simulink model "case5"  (R2024b)
settings: Solver=FixedStepAuto  StartTime=0  StopTime=1  FixedStep=1e-7  RelTol=1e-3
values from neighbouring files (symbols this model uses):
  SG_D_1_D = 0.01056    [IEEE9_case_parameters.m]    (also in case1_parameters.m; case2_parameters.m; case3_parameters.m; case4_parameters.m)
  SG_D_1_EnableSaturation = 0    [IEEE9_case_parameters.m]    (also in case1_parameters.m; case2_parameters.m; case3_parameters.m; case4_parameters.m)
  SG_D_1_f0 = 60    [IEEE9_case_parameters.m]    (also in case1_parameters.m; case2_parameters.m; case3_parameters.m; case4_parameters.m)
  SG_D_1_H = 7.5    [IEEE9_case_parameters.m]    (also in case1_parameters.m; case2_parameters.m; case3_parameters.m; case4_parameters.m)
  SG_D_1_K_A = 20    [IEEE9_case_parameters.m]    (also in case1_parameters.m; case2_parameters.m; case3_parameters.m; case4_parameters.m)
  SG_D_1_K_E = 1.000000e+1    (= 10)    [IEEE9_case_parameters.m]    (also in case1_parameters.m; case2_parameters.m; case3_parameters.m; case4_parameters.m)
  SG_D_1_K_F = 2.363    [IEEE9_case_parameters.m]    (also in case1_parameters.m; case2_parameters.m; case3_parameters.m; case4_parameters.m)
  SG_D_1_K_s = 0.5    [IEEE9_case_parameters.m]    (also in case1_parameters.m = 5; case2_parameters.m = 5; case3_parameters.m = 5; case4_parameters.m = 5)
  SG_D_1_R_a = 0.001088    [IEEE9_case_parameters.m]    (also in case1_parameters.m; case2_parameters.m; case3_parameters.m; case4_parameters.m)
  SG_D_1_S_A = 1    [IEEE9_case_parameters.m]    (also in case1_parameters.m; case2_parameters.m; case3_parameters.m; case4_parameters.m)
  SG_D_1_S_B = 0.103    [IEEE9_case_parameters.m]    (also in case1_parameters.m; case2_parameters.m; case3_parameters.m; case4_parameters.m)
  SG_D_1_S_N = 10.659857    [IEEE9_case_parameters.m]    (also in case1_parameters.m; case2_parameters.m; case3_parameters.m; case4_parameters.m)
  SG_D_1_SpeedPara = 200    [IEEE9_case_parameters.m]    (also in case1_parameters.m; case2_parameters.m; case3_parameters.m; case4_parameters.m)
  SG_D_1_T_0 = 0.720173    [IEEE9_case_parameters.m]    (also in case1_parameters.m = 0.755522; case2_parameters.m = 0.808931; case3_parameters.m = 0.869402; case4_parameters.m = 0.729316)
  SG_D_1_T_1 = 0.3    [IEEE9_case_parameters.m]    (also in case1_parameters.m; case2_parameters.m; case3_parameters.m; case4_parameters.m)
  SG_D_1_T_2 = 0.05    [IEEE9_case_parameters.m]    (also in case1_parameters.m; case2_parameters.m; case3_parameters.m; case4_parameters.m)
  SG_D_1_T_3 = 0.02    [IEEE9_case_parameters.m]    (also in case1_parameters.m; case2_parameters.m; case3_parameters.m; case4_parameters.m)
  SG_D_1_T_4 = 0.005    [IEEE9_case_parameters.m]    (also in case1_parameters.m; case2_parameters.m; case3_parameters.m; case4_parameters.m)
  SG_D_1_T_A = 0.02    [IEEE9_case_parameters.m]    (also in case1_parameters.m; case2_parameters.m; case3_parameters.m; case4_parameters.m)
  SG_D_1_T_dd = 8.000000e+0    (= 8)    [IEEE9_case_parameters.m]    (also in case1_parameters.m; case2_parameters.m; case3_parameters.m; case4_parameters.m)
  SG_D_1_T_ddd = 0.04    [IEEE9_case_parameters.m]    (also in case1_parameters.m; case2_parameters.m; case3_parameters.m; case4_parameters.m)
  SG_D_1_T_E = 0.314    [IEEE9_case_parameters.m]    (also in case1_parameters.m; case2_parameters.m; case3_parameters.m; case4_parameters.m)
  SG_D_1_T_F = 0.35    [IEEE9_case_parameters.m]    (also in case1_parameters.m; case2_parameters.m; case3_parameters.m; case4_parameters.m)
  SG_D_1_T_qd = 0.8    [IEEE9_case_parameters.m]    (also in case1_parameters.m; case2_parameters.m; case3_parameters.m; case4_parameters.m)
  SG_D_1_T_qdd = 0.02    [IEEE9_case_parameters.m]    (also in case1_parameters.m; case2_parameters.m; case3_parameters.m; case4_parameters.m)
  SG_D_1_T_speed = 0.1    [IEEE9_case_parameters.m]    (also in case1_parameters.m = 200; case2_parameters.m = 200; case3_parameters.m = 200; case4_parameters.m = 200)
  SG_D_1_T_w = 0.5    [IEEE9_case_parameters.m]    (also in case1_parameters.m; case2_parameters.m; case3_parameters.m; case4_parameters.m)
  SG_D_1_V_ref = 1.990276    [IEEE9_case_parameters.m]    (also in case1_parameters.m = 2.042296; case2_parameters.m = 2.051388; case3_parameters.m = 2.089584; case4_parameters.m = 2.01845)
  SG_D_1_w_ref = 376.991118    [IEEE9_case_parameters.m]    (also in case1_parameters.m; case2_parameters.m; case3_parameters.m; case4_parameters.m)
  SG_D_1_wb = 6.000000e+1    (= 60)    [IEEE9_case_parameters.m]    (also in case1_parameters.m; case2_parameters.m; case3_parameters.m; case4_parameters.m)
  SG_D_1_x_d = 1.9    [IEEE9_case_parameters.m]    (also in case1_parameters.m; case2_parameters.m; case3_parameters.m; case4_parameters.m)
  SG_D_1_x_dd = 0.302    [IEEE9_case_parameters.m]    (also in case1_parameters.m; case2_parameters.m; case3_parameters.m; case4_parameters.m)
  SG_D_1_x_ddd = 0.204    [IEEE9_case_parameters.m]    (also in case1_parameters.m; case2_parameters.m; case3_parameters.m; case4_parameters.m)
  SG_D_1_x_l = 0.05    [IEEE9_case_parameters.m]    (also in case1_parameters.m; case2_parameters.m; case3_parameters.m; case4_parameters.m)
  SG_D_1_x_q = 1.3    [IEEE9_case_parameters.m]    (also in case1_parameters.m; case2_parameters.m; case3_parameters.m; case4_parameters.m)
  SG_D_1_x_qd = 0.5    [IEEE9_case_parameters.m]    (also in case1_parameters.m; case2_parameters.m; case3_parameters.m; case4_parameters.m)
  SG_D_1_x_qdd = 0.3    [IEEE9_case_parameters.m]    (also in case1_parameters.m; case2_parameters.m; case3_parameters.m; case4_parameters.m)
  SG_D_2_D = 0.02    [IEEE9_case_parameters.m]    (also in case1_parameters.m; case2_parameters.m; case3_parameters.m; case4_parameters.m)
  SG_D_2_EnableSaturation = 0    [IEEE9_case_parameters.m]    (also in case1_parameters.m; case2_parameters.m; case3_parameters.m; case4_parameters.m)
  SG_D_2_f0 = 60    [IEEE9_case_parameters.m]    (also in case1_parameters.m; case2_parameters.m; case3_parameters.m; case4_parameters.m)
  SG_D_2_H = 8.000000e+0    (= 8)    [IEEE9_case_parameters.m]    (also in case1_parameters.m; case2_parameters.m; case3_parameters.m; case4_parameters.m)
  SG_D_2_K_A = 20    [IEEE9_case_parameters.m]    (also in case1_parameters.m; case2_parameters.m; case3_parameters.m; case4_parameters.m)
  SG_D_2_K_E = 1.000000e+1    (= 10)    [IEEE9_case_parameters.m]    (also in case1_parameters.m; case2_parameters.m; case3_parameters.m; case4_parameters.m)
  SG_D_2_K_F = 2.363    [IEEE9_case_parameters.m]    (also in case1_parameters.m; case2_parameters.m; case3_parameters.m; case4_parameters.m)
  SG_D_2_K_s = 0.5    [IEEE9_case_parameters.m]    (also in case1_parameters.m = 4; case2_parameters.m = 4; case3_parameters.m = 4; case4_parameters.m = 4)
  SG_D_2_R_a = 0.001088    [IEEE9_case_parameters.m]    (also in case1_parameters.m; case2_parameters.m; case3_parameters.m; case4_parameters.m)
  SG_D_2_S_A = 1    [IEEE9_case_parameters.m]    (also in case1_parameters.m; case2_parameters.m; case3_parameters.m; case4_parameters.m)
  SG_D_2_S_B = 0.103    [IEEE9_case_parameters.m]    (also in case1_parameters.m; case2_parameters.m; case3_parameters.m; case4_parameters.m)
  SG_D_2_S_N = 10.659857    [IEEE9_case_parameters.m]    (also in case1_parameters.m; case2_parameters.m; case3_parameters.m; case4_parameters.m)
  SG_D_2_SpeedPara = 200    [IEEE9_case_parameters.m]    (also in case1_parameters.m; case2_parameters.m; case3_parameters.m; case4_parameters.m)
  SG_D_2_T_0 = 1.632913    [IEEE9_case_parameters.m]    (also in case1_parameters.m = 1.632925; case2_parameters.m = 1.632915; case3_parameters.m = 1.632914; case4_parameters.m = 1.632927)
  SG_D_2_T_1 = 0.2    [IEEE9_case_parameters.m]    (also in case1_parameters.m; case2_parameters.m; case3_parameters.m; case4_parameters.m)
  SG_D_2_T_2 = 0.05    [IEEE9_case_parameters.m]    (also in case1_parameters.m; case2_parameters.m; case3_parameters.m; case4_parameters.m)
  SG_D_2_T_3 = 0.02    [IEEE9_case_parameters.m]    (also in case1_parameters.m; case2_parameters.m; case3_parameters.m; case4_parameters.m)
  SG_D_2_T_4 = 0.005    [IEEE9_case_parameters.m]    (also in case1_parameters.m; case2_parameters.m; case3_parameters.m; case4_parameters.m)
  SG_D_2_T_A = 0.02    [IEEE9_case_parameters.m]    (also in case1_parameters.m; case2_parameters.m; case3_parameters.m; case4_parameters.m)
  SG_D_2_T_dd = 7.9    [IEEE9_case_parameters.m]    (also in case1_parameters.m; case2_parameters.m; case3_parameters.m; case4_parameters.m)
  SG_D_2_T_ddd = 0.04    [IEEE9_case_parameters.m]    (also in case1_parameters.m; case2_parameters.m; case3_parameters.m; case4_parameters.m)
  SG_D_2_T_E = 0.314    [IEEE9_case_parameters.m]    (also in case1_parameters.m; case2_parameters.m; case3_parameters.m; case4_parameters.m)
  SG_D_2_T_F = 0.35    [IEEE9_case_parameters.m]    (also in case1_parameters.m; case2_parameters.m; case3_parameters.m; case4_parameters.m)
  SG_D_2_T_qd = 0.8    [IEEE9_case_parameters.m]    (also in case1_parameters.m; case2_parameters.m; case3_parameters.m; case4_parameters.m)
  SG_D_2_T_qdd = 0.015    [IEEE9_case_parameters.m]    (also in case1_parameters.m; case2_parameters.m; case3_parameters.m; case4_parameters.m)
  SG_D_2_T_speed = 0.1    [IEEE9_case_parameters.m]    (also in case1_parameters.m = 150; case2_parameters.m = 150; case3_parameters.m = 150; case4_parameters.m = 150)
  SG_D_2_T_w = 0.35    [IEEE9_case_parameters.m]    (also in case1_parameters.m; case2_parameters.m; case3_parameters.m; case4_parameters.m)
  SG_D_2_V_ref = 2.58547    [IEEE9_case_parameters.m]    (also in case1_parameters.m = 2.597896; case2_parameters.m = 2.587136; case3_parameters.m = 2.586042; case4_parameters.m = 2.599679)
  SG_D_2_w_ref = 376.991118    [IEEE9_case_parameters.m]    (also in case1_parameters.m; case2_parameters.m; case3_parameters.m; case4_parameters.m)
  SG_D_2_wb = 6.000000e+1    (= 60)    [IEEE9_case_parameters.m]    (also in case1_parameters.m; case2_parameters.m; case3_parameters.m; case4_parameters.m)
  SG_D_2_x_d = 1.8    [IEEE9_case_parameters.m]    (also in case1_parameters.m; case2_parameters.m; case3_parameters.m; case4_parameters.m)
  SG_D_2_x_dd = 0.302    [IEEE9_case_parameters.m]    (also in case1_parameters.m; case2_parameters.m; case3_parameters.m; case4_parameters.m)
  SG_D_2_x_ddd = 0.204    [IEEE9_case_parameters.m]    (also in case1_parameters.m; case2_parameters.m; case3_parameters.m; case4_parameters.m)
  SG_D_2_x_l = 0.05    [IEEE9_case_parameters.m]    (also in case1_parameters.m; case2_parameters.m; case3_parameters.m; case4_parameters.m)
  SG_D_2_x_q = 1.25    [IEEE9_case_parameters.m]    (also in case1_parameters.m; case2_parameters.m; case3_parameters.m; case4_parameters.m)
  SG_D_2_x_qd = 0.5    [IEEE9_case_parameters.m]    (also in case1_parameters.m; case2_parameters.m; case3_parameters.m; case4_parameters.m)
  SG_D_2_x_qdd = 0.3    [IEEE9_case_parameters.m]    (also in case1_parameters.m; case2_parameters.m; case3_parameters.m; case4_parameters.m)
  SG_D_3_D = 0.02    [IEEE9_case_parameters.m]    (also in case1_parameters.m; case2_parameters.m; case3_parameters.m; case4_parameters.m)
  SG_D_3_EnableSaturation = 0    [IEEE9_case_parameters.m]    (also in case1_parameters.m; case2_parameters.m; case3_parameters.m; case4_parameters.m)
  SG_D_3_f0 = 60    [IEEE9_case_parameters.m]    (also in case1_parameters.m; case2_parameters.m; case3_parameters.m; case4_parameters.m)
  SG_D_3_H = 7.7    [IEEE9_case_parameters.m]    (also in case1_parameters.m; case2_parameters.m; case3_parameters.m; case4_parameters.m)
  SG_D_3_K_A = 20    [IEEE9_case_parameters.m]    (also in case1_parameters.m; case2_parameters.m; case3_parameters.m; case4_parameters.m)
  SG_D_3_K_E = 1.000000e+1    (= 10)    [IEEE9_case_parameters.m]    (also in case1_parameters.m; case2_parameters.m; case3_parameters.m; case4_parameters.m)
  SG_D_3_K_F = 2.363    [IEEE9_case_parameters.m]    (also in case1_parameters.m; case2_parameters.m; case3_parameters.m; case4_parameters.m)
  SG_D_3_K_s = 0.2    [IEEE9_case_parameters.m]    (also in case1_parameters.m = 2; case2_parameters.m = 2; case3_parameters.m = 2; case4_parameters.m = 2)
  SG_D_3_R_a = 0.001088    [IEEE9_case_parameters.m]    (also in case1_parameters.m; case2_parameters.m; case3_parameters.m; case4_parameters.m)
  SG_D_3_S_A = 1    [IEEE9_case_parameters.m]    (also in case1_parameters.m; case2_parameters.m; case3_parameters.m; case4_parameters.m)
  SG_D_3_S_B = 0.103    [IEEE9_case_parameters.m]    (also in case1_parameters.m; case2_parameters.m; case3_parameters.m; case4_parameters.m)
  SG_D_3_S_N = 10.659857    [IEEE9_case_parameters.m]    (also in case1_parameters.m; case2_parameters.m; case3_parameters.m; case4_parameters.m)
  SG_D_3_SpeedPara = 200    [IEEE9_case_parameters.m]    (also in case1_parameters.m; case2_parameters.m; case3_parameters.m; case4_parameters.m)
  SG_D_3_T_0 = 0.850788    [IEEE9_case_parameters.m]    (also in case1_parameters.m = 0.850786; case2_parameters.m = 0.850787; case3_parameters.m; case4_parameters.m = 0.850786)
  SG_D_3_T_1 = 0.2    [IEEE9_case_parameters.m]    (also in case1_parameters.m; case2_parameters.m; case3_parameters.m; case4_parameters.m)
  SG_D_3_T_2 = 0.05    [IEEE9_case_parameters.m]    (also in case1_parameters.m; case2_parameters.m; case3_parameters.m; case4_parameters.m)
  SG_D_3_T_3 = 0.02    [IEEE9_case_parameters.m]    (also in case1_parameters.m; case2_parameters.m; case3_parameters.m; case4_parameters.m)
  SG_D_3_T_4 = 0.005    [IEEE9_case_parameters.m]    (also in case1_parameters.m; case2_parameters.m; case3_parameters.m; case4_parameters.m)
  SG_D_3_T_A = 0.02    [IEEE9_case_parameters.m]    (also in case1_parameters.m; case2_parameters.m; case3_parameters.m; case4_parameters.m)
  SG_D_3_T_dd = 8.1    [IEEE9_case_parameters.m]    (also in case1_parameters.m; case2_parameters.m; case3_parameters.m; case4_parameters.m)
  SG_D_3_T_ddd = 0.04    [IEEE9_case_parameters.m]    (also in case1_parameters.m; case2_parameters.m; case3_parameters.m; case4_parameters.m)
  SG_D_3_T_E = 0.314    [IEEE9_case_parameters.m]    (also in case1_parameters.m; case2_parameters.m; case3_parameters.m; case4_parameters.m)
  SG_D_3_T_F = 0.35    [IEEE9_case_parameters.m]    (also in case1_parameters.m; case2_parameters.m; case3_parameters.m; case4_parameters.m)
  SG_D_3_T_qd = 0.8    [IEEE9_case_parameters.m]    (also in case1_parameters.m; case2_parameters.m; case3_parameters.m; case4_parameters.m)
  SG_D_3_T_qdd = 0.015    [IEEE9_case_parameters.m]    (also in case1_parameters.m; case2_parameters.m; case3_parameters.m; case4_parameters.m)
  SG_D_3_T_speed = 0.1    [IEEE9_case_parameters.m]    (also in case1_parameters.m = 180; case2_parameters.m = 180; case3_parameters.m = 180; case4_parameters.m = 180)
  SG_D_3_T_w = 0.4    [IEEE9_case_parameters.m]    (also in case1_parameters.m; case2_parameters.m; case3_parameters.m; case4_parameters.m)
  SG_D_3_V_ref = 1.892727    [IEEE9_case_parameters.m]    (also in case1_parameters.m = 1.906439; case2_parameters.m = 1.895535; case3_parameters.m = 1.892105; case4_parameters.m = 1.906598)
  SG_D_3_w_ref = 376.991118    [IEEE9_case_parameters.m]    (also in case1_parameters.m; case2_parameters.m; case3_parameters.m; case4_parameters.m)
  SG_D_3_wb = 6.000000e+1    (= 60)    [IEEE9_case_parameters.m]    (also in case1_parameters.m; case2_parameters.m; case3_parameters.m; case4_parameters.m)
  SG_D_3_x_d = 1.85    [IEEE9_case_parameters.m]    (also in case1_parameters.m; case2_parameters.m; case3_parameters.m; case4_parameters.m)
  SG_D_3_x_dd = 0.302    [IEEE9_case_parameters.m]    (also in case1_parameters.m; case2_parameters.m; case3_parameters.m; case4_parameters.m)
  SG_D_3_x_ddd = 0.204    [IEEE9_case_parameters.m]    (also in case1_parameters.m; case2_parameters.m; case3_parameters.m; case4_parameters.m)
  SG_D_3_x_l = 0.05    [IEEE9_case_parameters.m]    (also in case1_parameters.m; case2_parameters.m; case3_parameters.m; case4_parameters.m)
  SG_D_3_x_q = 1.2    [IEEE9_case_parameters.m]    (also in case1_parameters.m; case2_parameters.m; case3_parameters.m; case4_parameters.m)
  SG_D_3_x_qd = 0.5    [IEEE9_case_parameters.m]    (also in case1_parameters.m; case2_parameters.m; case3_parameters.m; case4_parameters.m)
  SG_D_3_x_qdd = 0.3    [IEEE9_case_parameters.m]    (also in case1_parameters.m; case2_parameters.m; case3_parameters.m; case4_parameters.m)
(part 4 of 12)

== system case5/AC_1/d_vq_bus_7_block ==
  note: d_vq_bus_7 in case5
      | $2106.09563369148\,\mathrm{iq}_{\mathrm{bus},7}-376.991118430775\,\mathrm{vd}_{\mathrm{bus},7}$
      | Automatically generated on 2025-10-31 19:13:58 .
  Alge_iq_bus_7_45bb2 : Inport
  State_vd_bus_7_3739f : Inport  Port=2
  Constant_2106.09563369148_ba6a5 : Constant  Value=2106.09563369148
  Constant_376.991118430775_2faa8 : Constant  Value=376.991118430775
  Product_6eb21 : Product
  Product_90d6e : Product
  Subtract_950c2 : Sum  Inputs=+-
  Blockout_d_vq_bus_7_12864 : Outport
  wires:
  Constant_2106.09563369148_ba6a5/1 -> Product_6eb21/1
  Product_90d6e/1 -> Subtract_950c2/2
  Alge_iq_bus_7_45bb2/1 -> Product_6eb21/2
  Constant_376.991118430775_2faa8/1 -> Product_90d6e/1
  Subtract_950c2/1 -> Blockout_d_vq_bus_7_12864/1
  State_vd_bus_7_3739f/1 -> Product_90d6e/2
  Product_6eb21/1 -> Subtract_950c2/1

== system case5/AC_1/d_vq_bus_8_block ==
  note: d_vq_bus_8 in case5
      | $1657.10381727813\,\mathrm{iq}_{\mathrm{bus},8}-376.991118430775\,\mathrm{vd}_{\mathrm{bus},8}$
      | Automatically generated on 2025-10-31 19:14:00 .
  Alge_iq_bus_8_1b1c2 : Inport
  State_vd_bus_8_d6cf7 : Inport  Port=2
  Constant_1657.10381727813_ee9d3 : Constant  Value=1657.10381727813
  Constant_376.991118430775_c08d9 : Constant  Value=376.991118430775
  Product_2c011 : Product
  Product_4bb21 : Product
  Subtract_80bfc : Sum  Inputs=+-
  Blockout_d_vq_bus_8_57dfd : Outport
  wires:
  Constant_1657.10381727813_ee9d3/1 -> Product_2c011/1
  Constant_376.991118430775_c08d9/1 -> Product_4bb21/1
  Alge_iq_bus_8_1b1c2/1 -> Product_2c011/2
  State_vd_bus_8_d6cf7/1 -> Product_4bb21/2
  Product_2c011/1 -> Subtract_80bfc/1
  Product_4bb21/1 -> Subtract_80bfc/2
  Subtract_80bfc/1 -> Blockout_d_vq_bus_8_57dfd/1

== system case5/AC_1/d_vq_bus_9_block ==
  note: d_vq_bus_9 in case5
      | $1564.27849971276\,\mathrm{iq}_{\mathrm{bus},9}-376.991118430775\,\mathrm{vd}_{\mathrm{bus},9}$
      | Automatically generated on 2025-10-31 19:14:02 .
  Alge_iq_bus_9_3d507 : Inport
  State_vd_bus_9_5d984 : Inport  Port=2
  Constant_1564.27849971276_97533 : Constant  Value=1564.27849971276
  Constant_376.991118430775_b4458 : Constant  Value=376.991118430775
  Product_0f672 : Product
  Product_b1dd5 : Product
  Subtract_083c6 : Sum  Inputs=+-
  Blockout_d_vq_bus_9_906de : Outport
  wires:
  Constant_1564.27849971276_97533/1 -> Product_0f672/1
  Constant_376.991118430775_b4458/1 -> Product_b1dd5/1
  Alge_iq_bus_9_3d507/1 -> Product_0f672/2
  State_vd_bus_9_5d984/1 -> Product_b1dd5/2
  Product_0f672/1 -> Subtract_083c6/1
  Product_b1dd5/1 -> Subtract_083c6/2
  Subtract_083c6/1 -> Blockout_d_vq_bus_9_906de/1

== system case5/AC_1/id_bus_1_block ==
  note: id_bus_1 in case5
      | $\mathrm{id}_{\mathrm{SG},D,1}-\mathrm{id}_{\mathrm{line},1,4}$
      | Automatically generated on 2025-10-31 19:14:43 .
  Input_id_SG_D_1_9c228 : Inport
  State_id_line_1_4_23de7 : Inport  Port=2
  Subtract_cb11a : Sum  Inputs=+-
  Blockout_id_bus_1_91a25 : Outport
  wires:
  Input_id_SG_D_1_9c228/1 -> Subtract_cb11a/1
  State_id_line_1_4_23de7/1 -> Subtract_cb11a/2
  Subtract_cb11a/1 -> Blockout_id_bus_1_91a25/1

== system case5/AC_1/id_bus_2_block ==
  note: id_bus_2 in case5
      | $\mathrm{id}_{\mathrm{SG},D,2}+\mathrm{id}_{\mathrm{line},8,2}$
      | Automatically generated on 2025-10-31 19:14:45 .
  Input_id_SG_D_2_cb453 : Inport
  State_id_line_8_2_49dbc : Inport  Port=2
  Add_a3873 : Sum
  Blockout_id_bus_2_c40f0 : Outport
  wires:
  Input_id_SG_D_2_cb453/1 -> Add_a3873/1
  State_id_line_8_2_49dbc/1 -> Add_a3873/2
  Add_a3873/1 -> Blockout_id_bus_2_c40f0/1

== system case5/AC_1/id_bus_3_block ==
  note: id_bus_3 in case5
      | $\mathrm{id}_{\mathrm{SG},D,3}-\mathrm{id}_{\mathrm{line},3,6}$
      | Automatically generated on 2025-10-31 19:14:48 .
  Input_id_SG_D_3_99f83 : Inport
  State_id_line_3_6_1713b : Inport  Port=2
  Subtract_3e534 : Sum  Inputs=+-
  Blockout_id_bus_3_bec8f : Outport
  wires:
  Input_id_SG_D_3_99f83/1 -> Subtract_3e534/1
  State_id_line_3_6_1713b/1 -> Subtract_3e534/2
  Subtract_3e534/1 -> Blockout_id_bus_3_bec8f/1

== system case5/AC_1/id_bus_4_block ==
  note: id_bus_4 in case5
      | $\mathrm{id}_{\mathrm{line},1,4}-\mathrm{id}_{\mathrm{line},4,5}+\mathrm{id}_{\mathrm{line},9,4}$
      | Automatically generated on 2025-10-31 19:14:50 .
  State_id_line_1_4_47296 : Inport
  State_id_line_4_5_4344a : Inport  Port=2
  State_id_line_9_4_2502b : Inport  Port=3
  Add_be097 : Sum
  Subtract_45d26 : Sum  Inputs=+-
  Blockout_id_bus_4_70fca : Outport
  wires:
  State_id_line_9_4_2502b/1 -> Add_be097/2
  State_id_line_1_4_47296/1 -> Subtract_45d26/1
  State_id_line_4_5_4344a/1 -> Subtract_45d26/2
  Subtract_45d26/1 -> Add_be097/1
  Add_be097/1 -> Blockout_id_bus_4_70fca/1

== system case5/AC_1/id_bus_5_block ==
  note: id_bus_5 in case5
      | $\mathrm{id}_{\mathrm{line},4,5}-\mathrm{id}_{\mathrm{load},5}-\mathrm{id}_{\mathrm{line},5,6}$
      | Automatically generated on 2025-10-31 19:14:52 .
  State_id_load_5_d4ed3 : Inport
  State_id_line_4_5_425cc : Inport  Port=2
  State_id_line_5_6_e79c9 : Inport  Port=3
  Add_efccb : Sum
  Constant_-1_cbbea : Constant  Value=-1
  Product_350a7 : Product
  Subtract_95ac5 : Sum  Inputs=+-
  Blockout_id_bus_5_e7f75 : Outport
  wires:
  Subtract_95ac5/1 -> Blockout_id_bus_5_e7f75/1
  State_id_line_4_5_425cc/1 -> Add_efccb/2
  Constant_-1_cbbea/1 -> Product_350a7/1
  Add_efccb/1 -> Subtract_95ac5/1
  State_id_load_5_d4ed3/1 -> Product_350a7/2
  Product_350a7/1 -> Add_efccb/1
  State_id_line_5_6_e79c9/1 -> Subtract_95ac5/2

== system case5/AC_1/id_bus_6_block ==
  note: id_bus_6 in case5
      | $\mathrm{id}_{\mathrm{line},3,6}+\mathrm{id}_{\mathrm{line},5,6}-\mathrm{id}_{\mathrm{line},6,7}$
      | Automatically generated on 2025-10-31 19:14:54 .
  State_id_line_3_6_811b8 : Inport
  State_id_line_5_6_98abd : Inport  Port=2
  State_id_line_6_7_21130 : Inport  Port=3
  Add_d4af5 : Sum
  Subtract_01d0a : Sum  Inputs=+-
  Blockout_id_bus_6_b6b8c : Outport
  wires:
  State_id_line_6_7_21130/1 -> Subtract_01d0a/2
  State_id_line_3_6_811b8/1 -> Add_d4af5/1
  State_id_line_5_6_98abd/1 -> Add_d4af5/2
  Add_d4af5/1 -> Subtract_01d0a/1
  Subtract_01d0a/1 -> Blockout_id_bus_6_b6b8c/1

== system case5/AC_1/id_bus_7_block ==
  note: id_bus_7 in case5
      | $\mathrm{id}_{\mathrm{line},6,7}-\mathrm{id}_{\mathrm{load},7}-\mathrm{id}_{\mathrm{line},7,8}$
      | Automatically generated on 2025-10-31 19:14:56 .
  State_id_load_7_7bf08 : Inport
  State_id_line_6_7_06d30 : Inport  Port=2
  State_id_line_7_8_80602 : Inport  Port=3
  Add_eed5a : Sum
  Constant_-1_70b3b : Constant  Value=-1
  Product_29b3c : Product
  Subtract_43355 : Sum  Inputs=+-
  Blockout_id_bus_7_23be7 : Outport
  wires:
  Subtract_43355/1 -> Blockout_id_bus_7_23be7/1
  State_id_line_6_7_06d30/1 -> Add_eed5a/2
  Constant_-1_70b3b/1 -> Product_29b3c/1
  Add_eed5a/1 -> Subtract_43355/1
  State_id_load_7_7bf08/1 -> Product_29b3c/2
  Product_29b3c/1 -> Add_eed5a/1
  State_id_line_7_8_80602/1 -> Subtract_43355/2

== system case5/AC_1/id_bus_8_block ==
  note: id_bus_8 in case5
      | $\mathrm{id}_{\mathrm{line},7,8}-\mathrm{id}_{\mathrm{line},8,2}-\mathrm{id}_{\mathrm{line},8,9}$
      | Automatically generated on 2025-10-31 19:14:58 .
  State_id_line_7_8_30e25 : Inport
  State_id_line_8_2_6b72a : Inport  Port=2
  State_id_line_8_9_be4b7 : Inport  Port=3
  Subtract_2ee3c : Sum  Inputs=+-
  Subtract_46dea : Sum  Inputs=+-
  Blockout_id_bus_8_10175 : Outport
  wires:
  State_id_line_8_9_be4b7/1 -> Subtract_2ee3c/2
  State_id_line_7_8_30e25/1 -> Subtract_46dea/1
  State_id_line_8_2_6b72a/1 -> Subtract_46dea/2
  Subtract_46dea/1 -> Subtract_2ee3c/1
  Subtract_2ee3c/1 -> Blockout_id_bus_8_10175/1

== system case5/AC_1/id_bus_9_block ==
  note: id_bus_9 in case5
      | $\mathrm{id}_{\mathrm{line},8,9}-\mathrm{id}_{\mathrm{load},9}-\mathrm{id}_{\mathrm{line},9,4}$
      | Automatically generated on 2025-10-31 19:15:00 .
  State_id_load_9_599d3 : Inport
  State_id_line_8_9_6f7fd : Inport  Port=2
  State_id_line_9_4_83515 : Inport  Port=3
  Add_55017 : Sum
  Constant_-1_0a66a : Constant  Value=-1
  Product_dee9f : Product
  Subtract_f3c68 : Sum  Inputs=+-
  Blockout_id_bus_9_60bfe : Outport
  wires:
  Subtract_f3c68/1 -> Blockout_id_bus_9_60bfe/1
  State_id_line_8_9_6f7fd/1 -> Add_55017/2
  Constant_-1_0a66a/1 -> Product_dee9f/1
  Add_55017/1 -> Subtract_f3c68/1
  State_id_load_9_599d3/1 -> Product_dee9f/2
  Product_dee9f/1 -> Add_55017/1
  State_id_line_9_4_83515/1 -> Subtract_f3c68/2

== system case5/AC_1/iq_bus_1_block ==
  note: iq_bus_1 in case5
      | $\mathrm{iq}_{\mathrm{SG},D,1}-\mathrm{iq}_{\mathrm{line},1,4}$
      | Automatically generated on 2025-10-31 19:14:43 .
  Input_iq_SG_D_1_08f14 : Inport
  State_iq_line_1_4_e657d : Inport  Port=2
  Subtract_aca48 : Sum  Inputs=+-
  Blockout_iq_bus_1_da657 : Outport
  wires:
  Input_iq_SG_D_1_08f14/1 -> Subtract_aca48/1
  State_iq_line_1_4_e657d/1 -> Subtract_aca48/2
  Subtract_aca48/1 -> Blockout_iq_bus_1_da657/1

== system case5/AC_1/iq_bus_2_block ==
  note: iq_bus_2 in case5
      | $\mathrm{iq}_{\mathrm{SG},D,2}+\mathrm{iq}_{\mathrm{line},8,2}$
      | Automatically generated on 2025-10-31 19:14:46 .
  Input_iq_SG_D_2_79eaf : Inport
  State_iq_line_8_2_2ed82 : Inport  Port=2
  Add_b955d : Sum
  Blockout_iq_bus_2_efb5b : Outport
  wires:
  Input_iq_SG_D_2_79eaf/1 -> Add_b955d/1
  State_iq_line_8_2_2ed82/1 -> Add_b955d/2
  Add_b955d/1 -> Blockout_iq_bus_2_efb5b/1

== system case5/AC_1/iq_bus_3_block ==
  note: iq_bus_3 in case5
      | $\mathrm{iq}_{\mathrm{SG},D,3}-\mathrm{iq}_{\mathrm{line},3,6}$
      | Automatically generated on 2025-10-31 19:14:49 .
  Input_iq_SG_D_3_679b5 : Inport
  State_iq_line_3_6_d3a99 : Inport  Port=2
  Subtract_36106 : Sum  Inputs=+-
  Blockout_iq_bus_3_3b6b3 : Outport
  wires:
  Input_iq_SG_D_3_679b5/1 -> Subtract_36106/1
  State_iq_line_3_6_d3a99/1 -> Subtract_36106/2
  Subtract_36106/1 -> Blockout_iq_bus_3_3b6b3/1

== system case5/AC_1/iq_bus_4_block ==
  note: iq_bus_4 in case5
      | $\mathrm{iq}_{\mathrm{line},1,4}-\mathrm{iq}_{\mathrm{line},4,5}+\mathrm{iq}_{\mathrm{line},9,4}$
      | Automatically generated on 2025-10-31 19:14:51 .
  State_iq_line_1_4_c5db2 : Inport
  State_iq_line_4_5_0f8d8 : Inport  Port=2
  State_iq_line_9_4_ed85c : Inport  Port=3
  Add_38c5e : Sum
  Subtract_8af62 : Sum  Inputs=+-
  Blockout_iq_bus_4_10eb1 : Outport
  wires:
  State_iq_line_1_4_c5db2/1 -> Subtract_8af62/1
  State_iq_line_4_5_0f8d8/1 -> Subtract_8af62/2
  Subtract_8af62/1 -> Add_38c5e/1
  State_iq_line_9_4_ed85c/1 -> Add_38c5e/2
  Add_38c5e/1 -> Blockout_iq_bus_4_10eb1/1

== system case5/AC_1/iq_bus_5_block ==
  note: iq_bus_5 in case5
      | $\mathrm{iq}_{\mathrm{line},4,5}-\mathrm{iq}_{\mathrm{load},5}-\mathrm{iq}_{\mathrm{line},5,6}$
      | Automatically generated on 2025-10-31 19:14:53 .
  State_iq_load_5_13280 : Inport
  State_iq_line_4_5_a44be : Inport  Port=2
  State_iq_line_5_6_a1b62 : Inport  Port=3
  Add_5db17 : Sum
  Constant_-1_aaef8 : Constant  Value=-1
  Product_d522c : Product
  Subtract_9f494 : Sum  Inputs=+-
  Blockout_iq_bus_5_0fe3b : Outport
  wires:
  Subtract_9f494/1 -> Blockout_iq_bus_5_0fe3b/1
  State_iq_line_4_5_a44be/1 -> Add_5db17/2
  Constant_-1_aaef8/1 -> Product_d522c/1
  State_iq_load_5_13280/1 -> Product_d522c/2
  Product_d522c/1 -> Add_5db17/1
  Add_5db17/1 -> Subtract_9f494/1
  State_iq_line_5_6_a1b62/1 -> Subtract_9f494/2

== system case5/AC_1/iq_bus_6_block ==
  note: iq_bus_6 in case5
      | $\mathrm{iq}_{\mathrm{line},3,6}+\mathrm{iq}_{\mathrm{line},5,6}-\mathrm{iq}_{\mathrm{line},6,7}$
      | Automatically generated on 2025-10-31 19:14:55 .
  State_iq_line_3_6_7b556 : Inport
  State_iq_line_5_6_5b4f1 : Inport  Port=2
  State_iq_line_6_7_a49c1 : Inport  Port=3
  Add_13273 : Sum
  Subtract_8ba3b : Sum  Inputs=+-
  Blockout_iq_bus_6_a4840 : Outport
  wires:
  State_iq_line_3_6_7b556/1 -> Add_13273/1
  State_iq_line_5_6_5b4f1/1 -> Add_13273/2
  Add_13273/1 -> Subtract_8ba3b/1
  State_iq_line_6_7_a49c1/1 -> Subtract_8ba3b/2
  Subtract_8ba3b/1 -> Blockout_iq_bus_6_a4840/1

== system case5/AC_1/iq_bus_7_block ==
  note: iq_bus_7 in case5
      | $\mathrm{iq}_{\mathrm{line},6,7}-\mathrm{iq}_{\mathrm{load},7}-\mathrm{iq}_{\mathrm{line},7,8}$
      | Automatically generated on 2025-10-31 19:14:57 .
  State_iq_load_7_fc531 : Inport
  State_iq_line_6_7_dc5b1 : Inport  Port=2
  State_iq_line_7_8_6f400 : Inport  Port=3
  Add_a821c : Sum
  Constant_-1_32323 : Constant  Value=-1
  Product_79aa5 : Product
  Subtract_fce44 : Sum  Inputs=+-
  Blockout_iq_bus_7_c0ccf : Outport
  wires:
  Subtract_fce44/1 -> Blockout_iq_bus_7_c0ccf/1
  State_iq_line_6_7_dc5b1/1 -> Add_a821c/2
  Constant_-1_32323/1 -> Product_79aa5/1
  State_iq_load_7_fc531/1 -> Product_79aa5/2
  Product_79aa5/1 -> Add_a821c/1
  Add_a821c/1 -> Subtract_fce44/1
  State_iq_line_7_8_6f400/1 -> Subtract_fce44/2

== system case5/AC_1/iq_bus_8_block ==
  note: iq_bus_8 in case5
      | $\mathrm{iq}_{\mathrm{line},7,8}-\mathrm{iq}_{\mathrm{line},8,2}-\mathrm{iq}_{\mathrm{line},8,9}$
      | Automatically generated on 2025-10-31 19:14:59 .
  State_iq_line_7_8_27acc : Inport
  State_iq_line_8_2_45289 : Inport  Port=2
  State_iq_line_8_9_6eee5 : Inport  Port=3
  Subtract_1e44b : Sum  Inputs=+-
  Subtract_9d086 : Sum  Inputs=+-
  Blockout_iq_bus_8_30cc3 : Outport
  wires:
  State_iq_line_7_8_27acc/1 -> Subtract_1e44b/1
  State_iq_line_8_2_45289/1 -> Subtract_1e44b/2
  Subtract_1e44b/1 -> Subtract_9d086/1
  State_iq_line_8_9_6eee5/1 -> Subtract_9d086/2
  Subtract_9d086/1 -> Blockout_iq_bus_8_30cc3/1

== system case5/AC_1/iq_bus_9_block ==
  note: iq_bus_9 in case5
      | $\mathrm{iq}_{\mathrm{line},8,9}-\mathrm{iq}_{\mathrm{load},9}-\mathrm{iq}_{\mathrm{line},9,4}$
      | Automatically generated on 2025-10-31 19:15:01 .
  State_iq_load_9_e5f0b : Inport
  State_iq_line_8_9_086c3 : Inport  Port=2
  State_iq_line_9_4_06703 : Inport  Port=3
  Add_b2070 : Sum
  Constant_-1_91222 : Constant  Value=-1
  Product_39c09 : Product
  Subtract_641fc : Sum  Inputs=+-
  Blockout_iq_bus_9_35095 : Outport
  wires:
  Subtract_641fc/1 -> Blockout_iq_bus_9_35095/1
  State_iq_line_8_9_086c3/1 -> Add_b2070/2
  Constant_-1_91222/1 -> Product_39c09/1
  State_iq_load_9_e5f0b/1 -> Product_39c09/2
  Product_39c09/1 -> Add_b2070/1
  Add_b2070/1 -> Subtract_641fc/1
  State_iq_line_9_4_06703/1 -> Subtract_641fc/2

== system case5/AC_1/vd_bus_1_out_block ==
  note: vd_bus_1_out in case5
      | $\mathrm{vd}_{\mathrm{bus},1}$
      | Automatically generated on 2025-10-31 19:14:42 .
  State_vd_bus_1_d8d67 : Inport
  Blockout_vd_bus_1_out_40167 : Outport
  wires:
  State_vd_bus_1_d8d67/1 -> Blockout_vd_bus_1_out_40167/1

== system case5/AC_1/vd_bus_2_out_block ==
  note: vd_bus_2_out in case5
      | $\mathrm{vd}_{\mathrm{bus},2}$
      | Automatically generated on 2025-10-31 19:14:43 .
  State_vd_bus_2_9b70b : Inport
  Blockout_vd_bus_2_out_4bf4d : Outport
  wires:
  State_vd_bus_2_9b70b/1 -> Blockout_vd_bus_2_out_4bf4d/1

== system case5/AC_1/vd_bus_3_out_block ==
  note: vd_bus_3_out in case5
      | $\mathrm{vd}_{\mathrm{bus},3}$
      | Automatically generated on 2025-10-31 19:14:47 .
  State_vd_bus_3_3d199 : Inport
  Blockout_vd_bus_3_out_7cfd2 : Outport
  wires:
  State_vd_bus_3_3d199/1 -> Blockout_vd_bus_3_out_7cfd2/1

== system case5/AC_1/vq_bus_1_out_block ==
  note: vq_bus_1_out in case5
      | $\mathrm{vq}_{\mathrm{bus},1}$
      | Automatically generated on 2025-10-31 19:14:43 .
  State_vq_bus_1_cd4b3 : Inport
  Blockout_vq_bus_1_out_208d9 : Outport
  wires:
  State_vq_bus_1_cd4b3/1 -> Blockout_vq_bus_1_out_208d9/1

== system case5/AC_1/vq_bus_2_out_block ==
  note: vq_bus_2_out in case5
      | $\mathrm{vq}_{\mathrm{bus},2}$
      | Automatically generated on 2025-10-31 19:14:44 .
  State_vq_bus_2_2533a : Inport
  Blockout_vq_bus_2_out_5d720 : Outport
  wires:
  State_vq_bus_2_2533a/1 -> Blockout_vq_bus_2_out_5d720/1

== system case5/AC_1/vq_bus_3_out_block ==
  note: vq_bus_3_out in case5
      | $\mathrm{vq}_{\mathrm{bus},3}$
      | Automatically generated on 2025-10-31 19:14:48 .
  State_vq_bus_3_9de4a : Inport
  Blockout_vq_bus_3_out_e2cb2 : Outport
  wires:
  State_vq_bus_3_9de4a/1 -> Blockout_vq_bus_3_out_e2cb2/1

== system case5/SG_D_1/T_e_SG_D_1_block ==
  note: T_e_SG_D_1 in case5
      | $-\frac{\psi _{d,\mathrm{SG},D,1}\,\left(\psi _{q,\mathrm{SG},D,1}+\frac{\psi _{\mathrm{gq},\mathrm{SG},D,1}\,\left(x_{l}-x_{\mathrm{qdd}}\right)}{x_{l}-x_{\mathrm{qd}}}+\frac{\psi _{\mathrm{kq},\mathrm{SG},D,1}\,\left(x_{\mathrm{qd}}-x_{\mathrm{qdd}}\right)}{x_{l}-x_{\mathrm{qd}}}\right)}{x_{\mathrm{qdd}}}-\frac{\psi _{q,\mathrm{SG},D,1}\,\left(\frac{\psi _{\mathrm{1d},\mathrm{SG},D,1}\,\left(x_{\mathrm{dd}}-x_{\mathrm{ddd}}\right)}{x_{\mathrm{dd}}-x_{l}}-\psi _{d,\mathrm{SG},D,1}+\frac{\psi _{\mathrm{fd},\mathrm{SG},D,1}\,\left(x_{\mathrm{ddd}}-x_{l}\right)}{x_{\mathrm{dd}}-x_{l}}\right)}{x_{\mathrm{ddd}}}$
      | Automatically generated on 2025-10-31 19:10:40 .
  State_psi_d_SG_D_1_90645 : Inport
  State_psi_gq_SG_D_1_f0c91 : Inport  Port=2
  State_psi_kq_SG_D_1_a4a45 : Inport  Port=3
  State_psi_q_SG_D_1_cd1a7 : Inport  Port=4
  State_psi_q_SG_D_1_ce309 : Inport  Port=5
  State_psi_1d_SG_D_1_a3712 : Inport  Port=6
  State_psi_d_SG_D_1_8fbb1 : Inport  Port=7
  State_psi_fd_SG_D_1_11963 : Inport  Port=8
  Add_296ff : Sum
  Add_2a107 : Sum
  Add_2a2c1 : Sum
  Add_6cfcc : Sum
  Add_73ed4 : Sum
  Add_91617 : Sum
  Constant_-1_5b1ac : Constant  Value=-1
  Constant_-1_7cf8b : Constant  Value=-1
  Constant_-1_9b6ec : Constant  Value=-1
  Constant_-1_bbbe6 : Constant  Value=-1
  Constant_-1_ccaec : Constant  Value=-1
  Constant_x_dd_06fe6 : Constant  Value=x_dd
  Constant_x_dd_113b9 : Constant  Value=x_dd
  Constant_x_dd_aee66 : Constant  Value=x_dd
  Constant_x_ddd_0bf25 : Constant  Value=x_ddd
  Constant_x_ddd_aec0d : Constant  Value=x_ddd
  Constant_x_ddd_ed060 : Constant  Value=x_ddd
  Constant_x_l_0bcad : Constant  Value=x_l
  Constant_x_l_547c2 : Constant  Value=x_l
  Constant_x_l_708f5 : Constant  Value=x_l
  Constant_x_l_89317 : Constant  Value=x_l
  Constant_x_l_a351c : Constant  Value=x_l
  Constant_x_l_f42d2 : Constant  Value=x_l
  Constant_x_qd_83f59 : Constant  Value=x_qd
  Constant_x_qd_8a4e7 : Constant  Value=x_qd
  Constant_x_qd_ab7f5 : Constant  Value=x_qd
  Constant_x_qdd_0f9c8 : Constant  Value=x_qdd
  Constant_x_qdd_8e02c : Constant  Value=x_qdd
  Constant_x_qdd_b2075 : Constant  Value=x_qdd
  Divide_06796 : Product  Inputs=*/
  Divide_0d780 : Product  Inputs=*/
  Divide_15430 : Product  Inputs=*/
  Divide_a5e25 : Product  Inputs=*/
  Divide_b797e : Product  Inputs=*/
  Divide_d10b9 : Product  Inputs=*/
  Product_02d3f : Product
  Product_1dacb : Product
  Product_28c39 : Product
  Product_3b41d : Product
  Product_4f565 : Product
  Product_5bf39 : Product
  Product_60cd8 : Product
  Product_6a88a : Product
  Product_a174c : Product
  Product_a56f6 : Product
  Product_d1e90 : Product
  Subtract_0efda : Sum  Inputs=+-
  Subtract_17d72 : Sum  Inputs=+-
  Subtract_31e39 : Sum  Inputs=+-
  Subtract_5349a : Sum  Inputs=+-
  Subtract_a0433 : Sum  Inputs=+-
  Subtract_b4079 : Sum  Inputs=+-
  Subtract_dacee : Sum  Inputs=+-
  Blockout_T_e_SG_D_1_47b6a : Outport
  wires:
  Product_60cd8/1 -> Divide_d10b9/1
  Product_a174c/1 -> Add_296ff/1
  Divide_d10b9/1 -> Subtract_17d72/1
  Constant_-1_5b1ac/1 -> Product_a174c/1
  Constant_x_l_89317/1 -> Product_a174c/2
  Constant_x_qdd_b2075/1 -> Add_296ff/2
  Constant_x_qd_ab7f5/1 -> Subtract_31e39/1
  Constant_-1_7cf8b/1 -> Product_6a88a/1
  Constant_x_qdd_8e02c/1 -> Divide_06796/2
  Constant_x_qdd_0f9c8/1 -> Subtract_31e39/2
  State_psi_q_SG_D_1_ce309/1 -> Product_5bf39/1
  Constant_x_dd_06fe6/1 -> Subtract_0efda/1
  Constant_x_l_a351c/1 -> Product_6a88a/2
  Subtract_0efda/1 -> Product_4f565/2
  Constant_-1_bbbe6/1 -> Product_02d3f/1
  Constant_x_l_f42d2/1 -> Product_02d3f/2
  Subtract_5349a/1 -> Product_5bf39/2
  State_psi_q_SG_D_1_cd1a7/1 -> Add_6cfcc/2
  Constant_-1_9b6ec/1 -> Product_3b41d/1
  State_psi_1d_SG_D_1_a3712/1 -> Product_3b41d/2
  Constant_x_ddd_ed060/1 -> Subtract_0efda/2
  State_psi_gq_SG_D_1_f0c91/1 -> Product_60cd8/1
  Add_296ff/1 -> Product_60cd8/2
  Product_6a88a/1 -> Add_73ed4/1
  Product_d1e90/1 -> Product_28c39/1
  Constant_x_qd_8a4e7/1 -> Add_73ed4/2
  Product_4f565/1 -> Divide_a5e25/1
  State_psi_kq_SG_D_1_a4a45/1 -> Product_1dacb/1
  Add_73ed4/1 -> Divide_d10b9/2
  Subtract_31e39/1 -> Product_1dacb/2
  Product_02d3f/1 -> Add_2a107/1
  Constant_x_qd_83f59/1 -> Add_2a107/2
  Product_1dacb/1 -> Divide_0d780/1
  Product_3b41d/1 -> Product_4f565/1
  Constant_x_dd_113b9/1 -> Subtract_dacee/1
  Constant_x_l_708f5/1 -> Subtract_dacee/2
  Constant_x_ddd_aec0d/1 -> Subtract_b4079/1
  Product_5bf39/1 -> Divide_15430/1
  Constant_x_l_0bcad/1 -> Subtract_b4079/2
  Divide_06796/1 -> Add_2a2c1/1
  Product_28c39/1 -> Divide_06796/1
  Add_2a107/1 -> Divide_0d780/2
  Subtract_17d72/1 -> Add_6cfcc/1
  Divide_0d780/1 -> Subtract_17d72/2
  Subtract_dacee/1 -> Divide_a5e25/2
  State_psi_fd_SG_D_1_11963/1 -> Product_a56f6/1
  Constant_x_ddd_0bf25/1 -> Divide_15430/2
  Subtract_b4079/1 -> Product_a56f6/2
  Constant_x_dd_aee66/1 -> Subtract_a0433/1
  Constant_x_l_547c2/1 -> Subtract_a0433/2
  Divide_a5e25/1 -> Add_91617/1
  Add_91617/1 -> Subtract_5349a/1
  State_psi_d_SG_D_1_8fbb1/1 -> Add_91617/2
  Product_a56f6/1 -> Divide_b797e/1
  Subtract_a0433/1 -> Divide_b797e/2
  Constant_-1_ccaec/1 -> Product_d1e90/1
  State_psi_d_SG_D_1_90645/1 -> Product_d1e90/2
  Divide_b797e/1 -> Subtract_5349a/2
  Add_6cfcc/1 -> Product_28c39/2
  Divide_15430/1 -> Add_2a2c1/2
  Add_2a2c1/1 -> Blockout_T_e_SG_D_1_47b6a/1

== system case5/SG_D_1/d_E_fd_SG_D_1_block ==
  note: d_E_fd_SG_D_1 in case5
      | $\frac{V_{f,\mathrm{SG},D,1}-E_{\mathrm{fd},\mathrm{SG},D,1}\,K_{E}}{T_{E}}$
      | Automatically generated on 2025-10-31 19:10:23 .
  State_E_fd_SG_D_1_1c8d2 : Inport
  State_V_f_SG_D_1_f4af9 : Inport  Port=2
  Add_e2656 : Sum
  Constant_-1_fdcca : Constant  Value=-1
  Constant_K_E_19e1c : Constant  Value=K_E
  Constant_T_E_da837 : Constant  Value=T_E
  Divide_c706c : Product  Inputs=*/
  Product_88b08 : Product
  Product_ca6a0 : Product
  Blockout_d_E_fd_SG_D_1_5e902 : Outport
  wires:
  Add_e2656/1 -> Divide_c706c/1
  Constant_-1_fdcca/1 -> Product_88b08/1
  State_E_fd_SG_D_1_1c8d2/1 -> Product_88b08/2
  Product_88b08/1 -> Product_ca6a0/1
  Constant_K_E_19e1c/1 -> Product_ca6a0/2
  Product_ca6a0/1 -> Add_e2656/1
  Constant_T_E_da837/1 -> Divide_c706c/2
  State_V_f_SG_D_1_f4af9/1 -> Add_e2656/2
  Divide_c706c/1 -> Blockout_d_E_fd_SG_D_1_5e902/1

== system case5/SG_D_1/d_Px_1_SG_D_1_block ==
  note: d_Px_1_SG_D_1 in case5
      | $\frac{w_{\mathrm{SG},D,1}-2\,\pi \,f_{0}}{T_{w}}-\frac{\mathrm{Px}_{1,\mathrm{SG},D,1}}{T_{w}}$
      | Automatically generated on 2025-10-31 19:10:24 .
  State_Px_1_SG_D_1_50cb8 : Inport
  State_w_SG_D_1_3979b : Inport  Port=2
  Add_16fa8 : Sum
  Add_579a3 : Sum
  Constant_-1_50155 : Constant  Value=-1
  Constant_-2.0_7f14b : Constant  Value=-2.0
  Constant_T_w_28816 : Constant  Value=T_w
  Constant_T_w_3e2b6 : Constant  Value=T_w
  Constant_f0_42aec : Constant  Value=f0
  Constant_pi_6e749 : Constant  Value=pi
  Divide_0ec71 : Product  Inputs=*/
  Divide_2f682 : Product  Inputs=*/
  Product_26c2c : Product
  Product_47cc9 : Product
  Product_f9e69 : Product
  Blockout_d_Px_1_SG_D_1_85706 : Outport
  wires:
  Add_579a3/1 -> Blockout_d_Px_1_SG_D_1_85706/1
  Constant_-2.0_7f14b/1 -> Product_f9e69/1
  Product_26c2c/1 -> Divide_0ec71/1
  State_w_SG_D_1_3979b/1 -> Add_16fa8/2
  Constant_-1_50155/1 -> Product_26c2c/1
  Constant_f0_42aec/1 -> Product_47cc9/2
  Constant_pi_6e749/1 -> Product_f9e69/2
  Product_47cc9/1 -> Add_16fa8/1
  Product_f9e69/1 -> Product_47cc9/1
  State_Px_1_SG_D_1_50cb8/1 -> Product_26c2c/2
  Constant_T_w_28816/1 -> Divide_0ec71/2
  Add_16fa8/1 -> Divide_2f682/1
  Constant_T_w_3e2b6/1 -> Divide_2f682/2
  Divide_0ec71/1 -> Add_579a3/1
  Divide_2f682/1 -> Add_579a3/2

== system case5/SG_D_1/d_Px_2_SG_D_1_block ==
  note: d_Px_2_SG_D_1 in case5
      | $\frac{\mathrm{Px}_{1,\mathrm{SG},D,1}-T_{2}\,\left(\frac{\mathrm{Px}_{1,\mathrm{SG},D,1}}{T_{w}}-\frac{w_{\mathrm{SG},D,1}-2\,\pi \,f_{0}}{T_{w}}\right)}{T_{1}}-\frac{\mathrm{Px}_{2,\mathrm{SG},D,1}}{T_{1}}$
      | Automatically generated on 2025-10-31 19:10:26 .
  State_Px_2_SG_D_1_37bd3 : Inport
  State_Px_1_SG_D_1_cd8bf : Inport  Port=2
  State_Px_1_SG_D_1_d048c : Inport  Port=3
  State_w_SG_D_1_c572b : Inport  Port=4
  Add_9f59b : Sum
  Add_a5941 : Sum
  Add_dfb2f : Sum
  Add_e735e : Sum
  Constant_-1_1834d : Constant  Value=-1
  Constant_-1_f4374 : Constant  Value=-1
  Constant_-2.0_5c910 : Constant  Value=-2.0
  Constant_T_1_4217c : Constant  Value=T_1
  Constant_T_1_c720b : Constant  Value=T_1
  Constant_T_2_2cd4d : Constant  Value=T_2
  Constant_T_w_d0a78 : Constant  Value=T_w
  Constant_T_w_d20b2 : Constant  Value=T_w
  Constant_f0_76a3d : Constant  Value=f0
  Constant_pi_01338 : Constant  Value=pi
  Divide_29549 : Product  Inputs=*/
  Divide_32936 : Product  Inputs=*/
  Divide_78cfc : Product  Inputs=*/
  Divide_f7826 : Product  Inputs=*/
  Product_1039a : Product
  Product_6f45a : Product
  Product_89bf8 : Product
  Product_da595 : Product
  Product_e2e8f : Product
  Blockout_d_Px_2_SG_D_1_8a1c6 : Outport
  wires:
  Constant_-2.0_5c910/1 -> Product_89bf8/1
  State_w_SG_D_1_c572b/1 -> Add_dfb2f/2
  Constant_f0_76a3d/1 -> Product_e2e8f/2
  Constant_pi_01338/1 -> Product_89bf8/2
  Add_a5941/1 -> Product_6f45a/2
  Product_e2e8f/1 -> Add_dfb2f/1
  Divide_29549/1 -> Add_a5941/1
  Product_89bf8/1 -> Product_e2e8f/1
  Constant_T_w_d0a78/1 -> Divide_29549/2
  Constant_-1_1834d/1 -> Product_da595/1
  State_Px_1_SG_D_1_d048c/1 -> Product_da595/2
  Divide_32936/1 -> Add_9f59b/1
  Product_da595/1 -> Divide_29549/1
  Add_dfb2f/1 -> Divide_f7826/1
  Constant_T_w_d20b2/1 -> Divide_f7826/2
  Divide_f7826/1 -> Add_a5941/2
  Constant_T_2_2cd4d/1 -> Product_6f45a/1
  Constant_-1_f4374/1 -> Product_1039a/1
  State_Px_2_SG_D_1_37bd3/1 -> Product_1039a/2
  State_Px_1_SG_D_1_cd8bf/1 -> Add_e735e/1
  Product_6f45a/1 -> Add_e735e/2
  Add_e735e/1 -> Divide_78cfc/1
  Product_1039a/1 -> Divide_32936/1
  Constant_T_1_c720b/1 -> Divide_32936/2
  Constant_T_1_4217c/1 -> Divide_78cfc/2
  Divide_78cfc/1 -> Add_9f59b/2
  Add_9f59b/1 -> Blockout_d_Px_2_SG_D_1_8a1c6/1

== system case5/SG_D_1/d_Px_3_SG_D_1_block ==
  note: d_Px_3_SG_D_1 in case5
      | $\frac{\mathrm{Px}_{2,\mathrm{SG},D,1}+T_{4}\,\left(\frac{\mathrm{Px}_{1,\mathrm{SG},D,1}-T_{2}\,\left(\frac{\mathrm{Px}_{1,\mathrm{SG},D,1}}{T_{w}}-\frac{w_{\mathrm{SG},D,1}-2\,\pi \,f_{0}}{T_{w}}\right)}{T_{1}}-\frac{\mathrm{Px}_{2,\mathrm{SG},D,1}}{T_{1}}\right)}{T_{3}}-\frac{\mathrm{Px}_{3,\mathrm{SG},D,1}}{T_{3}}$
      | Automatically generated on 2025-10-31 19:10:28 .
  State_Px_3_SG_D_1_043cf : Inport
  State_Px_2_SG_D_1_d417b : Inport  Port=2
  State_Px_2_SG_D_1_7f631 : Inport  Port=3
  State_Px_1_SG_D_1_53e62 : Inport  Port=4
  State_Px_1_SG_D_1_57d0c : Inport  Port=5
  State_w_SG_D_1_734a8 : Inport  Port=6
  Add_1ac81 : Sum
  Add_1ad1a : Sum
  Add_4c0db : Sum
  Add_9edac : Sum
  Add_c45b5 : Sum
  Add_dd5e5 : Sum
  Constant_-1_9ec0e : Constant  Value=-1
  Constant_-1_afe8d : Constant  Value=-1
  Constant_-1_d8d83 : Constant  Value=-1
  Constant_-2.0_80182 : Constant  Value=-2.0
  Constant_T_1_de0c5 : Constant  Value=T_1
  Constant_T_1_f674a : Constant  Value=T_1
  Constant_T_2_b2ddb : Constant  Value=T_2
  Constant_T_3_730e9 : Constant  Value=T_3
  Constant_T_3_e30af : Constant  Value=T_3
  Constant_T_4_e6e30 : Constant  Value=T_4
  Constant_T_w_7af6a : Constant  Value=T_w
  Constant_T_w_9a4ac : Constant  Value=T_w
  Constant_f0_40338 : Constant  Value=f0
  Constant_pi_e2c38 : Constant  Value=pi
  Divide_30f1f : Product  Inputs=*/
  Divide_4992f : Product  Inputs=*/
  Divide_63744 : Product  Inputs=*/
  Divide_91ef0 : Product  Inputs=*/
  Divide_a749c : Product  Inputs=*/
  Divide_bda11 : Product  Inputs=*/
  Product_3cd94 : Product
  Product_59e7f : Product
  Product_7cc48 : Product
  Product_81345 : Product
  Product_bea79 : Product
  Product_caeb8 : Product
  Product_ece8e : Product
  Blockout_d_Px_3_SG_D_1_28941 : Outport
  wires:
  Constant_T_w_7af6a/1 -> Divide_a749c/2
  Constant_-1_9ec0e/1 -> Product_7cc48/1
  Add_1ad1a/1 -> Blockout_d_Px_3_SG_D_1_28941/1
  Constant_-2.0_80182/1 -> Product_ece8e/1
  State_w_SG_D_1_734a8/1 -> Add_dd5e5/2
  Constant_f0_40338/1 -> Product_caeb8/2
  State_Px_1_SG_D_1_57d0c/1 -> Product_7cc48/2
  Constant_pi_e2c38/1 -> Product_ece8e/2
  Product_caeb8/1 -> Add_dd5e5/1
  Product_ece8e/1 -> Product_caeb8/1
  Product_7cc48/1 -> Divide_a749c/1
  Divide_bda11/1 -> Add_1ad1a/1
  Constant_T_3_730e9/1 -> Divide_63744/2
  Add_dd5e5/1 -> Divide_4992f/1
  Constant_T_w_9a4ac/1 -> Divide_4992f/2
  Divide_a749c/1 -> Add_1ac81/1
  Divide_4992f/1 -> Add_1ac81/2
  Constant_-1_afe8d/1 -> Product_59e7f/1
  Constant_T_2_b2ddb/1 -> Product_3cd94/1
  Add_1ac81/1 -> Product_3cd94/2
  Constant_-1_d8d83/1 -> Product_bea79/1
  Divide_63744/1 -> Add_1ad1a/2
  Constant_T_3_e30af/1 -> Divide_bda11/2
  State_Px_2_SG_D_1_7f631/1 -> Product_bea79/2
  State_Px_1_SG_D_1_53e62/1 -> Add_c45b5/1
  Divide_30f1f/1 -> Add_9edac/1
  Product_3cd94/1 -> Add_c45b5/2
  Product_bea79/1 -> Divide_30f1f/1
  Product_59e7f/1 -> Divide_bda11/1
  Constant_T_1_de0c5/1 -> Divide_30f1f/2
  Add_c45b5/1 -> Divide_91ef0/1
  Constant_T_1_f674a/1 -> Divide_91ef0/2
  Divide_91ef0/1 -> Add_9edac/2
  Constant_T_4_e6e30/1 -> Product_81345/1
  Add_9edac/1 -> Product_81345/2
  State_Px_3_SG_D_1_043cf/1 -> Product_59e7f/2
  State_Px_2_SG_D_1_d417b/1 -> Add_4c0db/1
  Product_81345/1 -> Add_4c0db/2
  Add_4c0db/1 -> Divide_63744/1

== system case5/SG_D_1/d_R_f_SG_D_1_block ==
  note: d_R_f_SG_D_1 in case5
      | $-\frac{R_{f,\mathrm{SG},D,1}-\frac{E_{\mathrm{fd},\mathrm{SG},D,1}\,K_{F}}{T_{F}}}{T_{F}}$
      | Automatically generated on 2025-10-31 19:10:22 .
  State_E_fd_SG_D_1_563f1 : Inport
  State_R_f_SG_D_1_dffc8 : Inport  Port=2
  Constant_K_F_9f3a7 : Constant  Value=K_F
  Constant_T_F_13458 : Constant  Value=T_F
  Constant_T_F_94625 : Constant  Value=T_F
  Divide_0738a : Product  Inputs=*/
  Divide_29bc8 : Product  Inputs=*/
  Product_548fc : Product
  Subtract_edecb : Sum  Inputs=+-
  Blockout_d_R_f_SG_D_1_7e349 : Outport
  wires:
  Constant_K_F_9f3a7/1 -> Product_548fc/2
  Product_548fc/1 -> Divide_29bc8/1
  State_E_fd_SG_D_1_563f1/1 -> Product_548fc/1
  State_R_f_SG_D_1_dffc8/1 -> Subtract_edecb/2
  Constant_T_F_13458/1 -> Divide_29bc8/2
  Divide_29bc8/1 -> Subtract_edecb/1
  Divide_0738a/1 -> Blockout_d_R_f_SG_D_1_7e349/1
  Subtract_edecb/1 -> Divide_0738a/1
  Constant_T_F_94625/1 -> Divide_0738a/2

== system case5/SG_D_1/d_T_m_SG_D_1_block ==
  note: d_T_m_SG_D_1 in case5
      | $-\frac{T_{m,\mathrm{SG},D,1}-T_{0}+\frac{\mathrm{SpeedPara}\,\left(w_{\mathrm{SG},D,1}-w_{\mathrm{ref}}\right)}{2\,f_{0}\,\pi }}{T_{\mathrm{speed}}}$
      | Automatically generated on 2025-10-31 19:10:13 .
  State_w_SG_D_1_e7a7d : Inport
  State_T_m_SG_D_1_599df : Inport  Port=2
  Add_6541a : Sum
  Add_f612a : Sum
  Constant_-1_f8c5e : Constant  Value=-1
  Constant_2.0_15a3d : Constant  Value=2.0
  Constant_SpeedPara_ce7b8 : Constant  Value=SpeedPara
  Constant_T_0_c87fe : Constant  Value=T_0
  Constant_T_speed_53599 : Constant  Value=T_speed
  Constant_f0_e37ca : Constant  Value=f0
  Constant_pi_7efe2 : Constant  Value=pi
  Constant_w_ref_f27ab : Constant  Value=w_ref
  Divide_7a85b : Product  Inputs=*/
  Divide_ed911 : Product  Inputs=*/
  Product_0c6a9 : Product
  Product_1d411 : Product
  Product_6e9f6 : Product
  Product_aa12e : Product
  Subtract_3d345 : Sum  Inputs=+-
  Blockout_d_T_m_SG_D_1_655fc : Outport
  wires:
  Constant_-1_f8c5e/1 -> Product_1d411/1
  Constant_w_ref_f27ab/1 -> Add_f612a/2
  State_w_SG_D_1_e7a7d/1 -> Product_1d411/2
  Add_6541a/1 -> Subtract_3d345/1
  Add_f612a/1 -> Product_aa12e/2
  Product_1d411/1 -> Add_f612a/1
  Constant_2.0_15a3d/1 -> Product_6e9f6/1
  Constant_pi_7efe2/1 -> Product_6e9f6/2
  Constant_SpeedPara_ce7b8/1 -> Product_aa12e/1
  Product_6e9f6/1 -> Product_0c6a9/1
  Constant_f0_e37ca/1 -> Product_0c6a9/2
  Constant_T_speed_53599/1 -> Divide_ed911/2
  Product_aa12e/1 -> Divide_7a85b/1
  Product_0c6a9/1 -> Divide_7a85b/2
  Divide_7a85b/1 -> Add_6541a/1
  Constant_T_0_c87fe/1 -> Add_6541a/2
  State_T_m_SG_D_1_599df/1 -> Subtract_3d345/2
  Subtract_3d345/1 -> Divide_ed911/1
  Divide_ed911/1 -> Blockout_d_T_m_SG_D_1_655fc/1
